simulink model "TRAMI_STEP_AT_vehicle_ver01_R2018b"  (R2018b)
settings: Solver=ode8  StartTime=0  StopTime=end_time  FixedStep=sampling_time  RelTol=1e-3
StartFcn:
  | csvwrite('simstart.csv',1)
StopFcn:
  | csvwrite('simstop.csv',1)
values from neighbouring files (symbols this model uses):
  sampling_time = 0.0025    [METI_TRAMI_Thermal_ver01_Jmaab_PreLoad.m]
undefined symbols (not defined in the file or in its folder): ACC_D_Gain, ACC_I_Gain, ACC_P_Gain, ALT_CNT_ALT_OFF_RPM_HYS_rpm, ALT_CNT_ALT_ON_RPM_HYS_rpm, ALT_CNT_Alter_V_BASE_V, ALT_CNT_Alter_V_Kaisei_V, ALT_CNT_flag_disable_kaisei, ALT_CNT_V_Battely_Kudo_V, ALT_PNT_ALT_GDCurrent_A, ALT_PNT_ALT_GDVolt_V, ALT_PNT_Alter_limit_Current_V_table, ALT_PNT_Alter_limit_Current_V_table_x_rpm, ALT_PNT_Alter_trq_Nm_map, ALT_PNT_Alter_trq_Nm_map_x_rpm, ALT_PNT_Alter_trq_Nm_map_y_Current_A, ALT_PNT_Alter_trq_Nm_map_z_Volt_tgt_V, ALT_PNT_eta_pulley_alt, ALT_PNT_Gain_Alt_v_del, ALT_PNT_ratio_pulley_alt, ALT_PNT_Tau_Alternator_V_tgt_s, ALT_PNT_trq_alter_output_LL_Nm, BK_PNT_Pow_UL, BK_PNT_Tau_brake, Brk_LL, Brk_PGain, Brk_UL, BT_PNT_Lo_Capa_lo_batt_F, BT_PNT_Lo_ocv_SOC_lo_batt_OCV_V_table, BT_PNT_Lo_ocv_SOC_lo_batt_OCV_V_table_x_SOC, BT_PNT_Lo_R_lo_batt_ohm, BT_PNT_Lo_SOC_MAX_lo_batt, BT_PNT_Lo_SOC_MIN_lo_batt, BT_PNT_Lo_SOC_START_lo_batt, BT_PNT_Lo_V_start_ocv, Driver_Brake_Const1, Driver_Brake_Const3, Driver_Brake_Switch_Const2, Driver_Brk_sh, drivmode_ACC, drivmode_CONST, drivmode_GensokuKaisei, drivmode_GensokuRikko, drivmode_STOP, EL_PNT_R_bodyelec_lo_ohm, ENG_CNT_Accel_LL, ENG_CNT_Accel_UL, ENG_CNT_brak_idlestop, ENG_CNT_flag_idle_stop_exe, ENG_CNT_gain_p_per_isc, ENG_CNT_IdleSpeed_Const, ENG_CNT_omg_eng_fuelcut_rpm, ENG_CNT_per_isc_max, ENG_CNT_per_isc_min, ENG_CNT_per_throttle_fuelcut, ENG_CNT_per_throttle_isc_fb, ENG_CNT_Starter_timer_Const_s, ENG_CNT_Throttle_LL, ENG_CNT_Throttle_UL, ENG_CNT_V_car_idlestop_kmph ... (+29)
libraries: METI_Lib_vehicle_model x18, simulink x4, AZAPA_Lib_vehicle_model x1
(part 2 of 2)

== system TRAMI_STEP_AT_vehicle_ver01_R2018b/Vehicle/TR_PNT ==
  note: 転がり抵抗
  note: 並進⇔回転変換
  note: トルク⇔力変換
  note: omg (回転数rad/s) = v (車速m/s) / r (タイヤ半径(m))
  note: M (トルクNm) = F (力(N)） × r (タイヤ半径(m))
  note: 車両を動かす側が正
  note: 車両を動かす側が正
  trq_TR_in_Nm : Inport
  v_VL_PNT_mps : Inport  Port=2
  Constant2 : Constant  Value=1/tire_r
  Product5 : Product  RndMeth=Zero
  Product6 : Product  RndMeth=Zero
  Q_cal1 : METI_Lib_vehicle_model/P_cal  Commented=on  Type_energy=並進運動  Type_output_energy=出力  Power_name=Po_  t_Workspace_Name=TR_PNT_MECK_DN  P_VariableName=Po_TR_PNT_MECK_DN  Across_VariableName=v_TR_PNT_MECK_DN  Throgh_VariableName=F_TR_PNT_MECK_DN
      settings: SourceProductName=The database C:\Users\k-uekata\AppData\Roaming\MathWorks\MATLAB\R2018b\slblocks_master.db is locked, or a table in the database is locked. (database is locked)
  Q_cal2 : METI_Lib_vehicle_model/P_cal  Commented=on  Type_energy=回転運動  Type_output_energy=出力  Power_name=Po_  t_Workspace_Name=TR_PNT_MECK_UP  P_VariableName=Po_TR_PNT_MECK_UP  Across_VariableName=w_TR_PNT_MECK_UP  Throgh_VariableName=tq_TR_PNT_MECK_UP
      settings: SourceProductName=The database C:\Users\k-uekata\AppData\Roaming\MathWorks\MATLAB\R2018b\slblocks_master.db is locked, or a table in the database is locked. (database is locked)
  Sum2 : Sum  Inputs=-+|
  Terminator1 : Terminator  Commented=on
  Terminator2 : Terminator  Commented=on
  cal_roll_resi : METI_Lib_vehicle_model/vehicle_model/cal_roll_resi  Myu_tire=myu  Vehicle_Mass=M  Gravi_acc=g
      settings: SourceProductName=The database C:\Users\k-uekata\AppData\Roaming\MathWorks\MATLAB\R2018b\slblocks_master.db is locked, or a table in the database is locked. (database is locked)
  w_TR_PNT_radps : Outport
  f_TR_PNT_N : Outport  Port=2
  wires:
  Sum2/1 -> f_TR_PNT_N/1  "f_TR_PNT_N"
  cal_roll_resi/1 -> Sum2/1, Q_cal1/2
  Product6/1 -> Sum2/2, Q_cal2/2
  Q_cal1/1 -> Terminator1/1
  Constant2/1 -> Product6/1, Product5/2
  v_VL_PNT_mps/1 -> Product5/1, cal_roll_resi/1, Q_cal1/1, Q_cal2/1
  Q_cal2/1 -> Terminator2/1
  Product5/1 -> w_TR_PNT_radps/1  "w_TR_PNT_radps"
  trq_TR_in_Nm/1 -> Product6/2

== system TRAMI_STEP_AT_vehicle_ver01_R2018b/Vehicle/T_PT_TH_K ==
  From Workspace1 : FromWorkspace  VariableName=T_PT_TH_K  SampleTime=0  OutputAfterFinalValue=Holding final value
  Sum2 : Sum  Inputs=|++
  ℃⇒K : Constant  Value=273.15
  Out1 : Outport
  wires:
  From Workspace1/1 -> Sum2/1
  ℃⇒K/1 -> Sum2/2
  Sum2/1 -> Out1/1

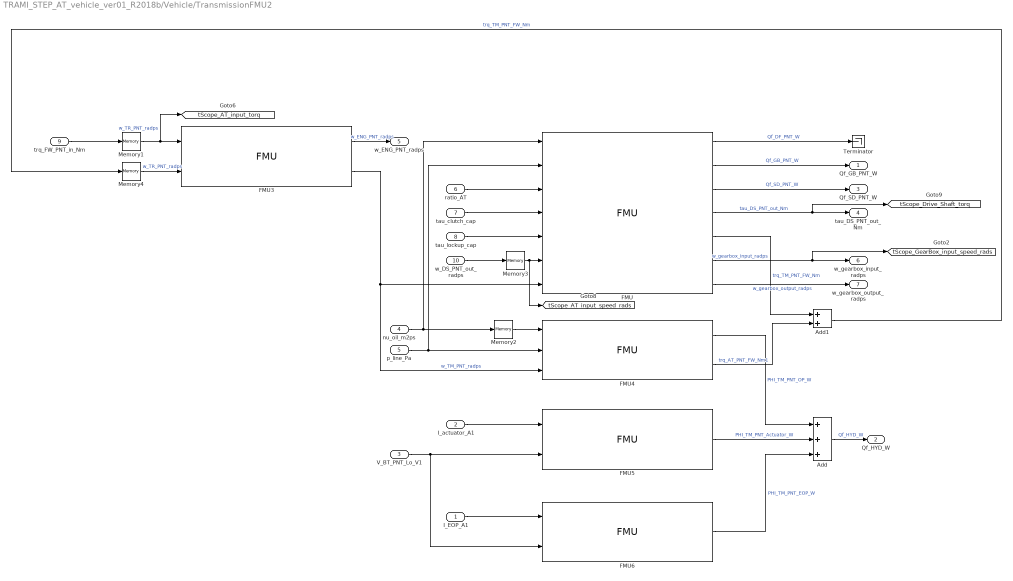
== system TRAMI_STEP_AT_vehicle_ver01_R2018b/Vehicle/TransmissionFMU2 ==
  I_EOP_A1 : Inport
  I_actuator_A1 : Inport  Port=2
  V_BT_PNT_Lo_V1 : Inport  Port=3
  nu_oil_m2ps : Inport  Port=4
  p_line_Pa : Inport  Port=5
  ratio_AT : Inport  Port=6
  tau_clutch_cap : Inport  Port=7
  tau_lockup_cap : Inport  Port=8
  trq_FW_PNT_in_Nm : Inport  Port=9
  w_DS_PNT_out_radps : Inport  Port=10
  Add : Sum  Inputs=+++
  Add1 : Sum
  FMU : FMU  FMUName=AtDsFmu.fmu  FMUMode=CoSimulation  minsamplestep=2.50000000000000000e-02  binfilename=DISABLED  mask(AtDsFmu [Co-Simulation, v2.0]){}
      mask Display: disp('AtDsFmu');
  FMU3 : FMU  FMUName=Flywheel.fmu  FMUMode=CoSimulation  Iwh=4.00000000000000000e-01  minsamplestep=2.50000000000000000e-02  binfilename=DISABLED  mask(Flywheel [Co-Simulation, v2.0]){}
      mask Display: disp('Flywheel');
  FMU4 : FMU  FMUName=OilPump.fmu  FMUMode=CoSimulation  Oil_Viscosity_Breakpoint_2=1.02000000000000000e-05  Oil_Viscosity_Breakpoint_3=1.69000000000000000e-05  Oil_Viscosity_Breakpoint_4=3.12000000000000000e-05  minsamplestep=2.50000000000000000e-02  binfilename=DISABLED  mask(OilPump [Co-Simulation, v2.0]){}
      mask Display: disp('OilPump');
  FMU5 : FMU  FMUName=ActuatorELoss.fmu  FMUMode=CoSimulation  minsamplestep=2.50000000000000000e-02  binfilename=DISABLED  mask(ActuatorELoss [Co-Simulation, v2.0]){}
      mask Display: disp('ActuatorELoss');
  FMU6 : FMU  FMUName=EOPELoss.fmu  FMUMode=CoSimulation  minsamplestep=2.50000000000000000e-02  binfilename=DISABLED  mask(EOPELoss [Co-Simulation, v2.0]){}
      mask Display: disp('EOPELoss');
  Memory{1..4} (4 alike) : Memory
  Terminator : Terminator
  Qf_GB_PNT_W : Outport
  Qf_HYD_W : Outport  Port=2
  Qf_SD_PNT_W : Outport  Port=3
  tau_DS_PNT_out_Nm : Outport  Port=4
  w_ENG_PNT_radps : Outport  Port=5
  w_gearbox_input_radps : Outport  Port=6
  w_gearbox_output_radps : Outport  Port=7
  tag scope: tScope_AT_input_speed_rads=global, tScope_AT_input_torq=global, tScope_Drive_Shaft_torq=global, tScope_GearBox_input_speed_rads=global
  wires:
  FMU3/1 -> w_ENG_PNT_radps/1  "w_ENG_PNT_radps"
  FMU5/1 -> Add/2  "PHI_TM_PNT_Actuator_W"
  FMU6/1 -> Add/3  "PHI_TM_PNT_EOP_W"
  FMU4/1 -> Add/1  "PHI_TM_PNT_OP_W"
  Add/1 -> Qf_HYD_W/1  "Qf_HYD_W"
  FMU4/2 -> Add1/2  "trq_AT_PNT_FW_Nm1"
  I_EOP_A1/1 -> FMU6/1
  I_actuator_A1/1 -> FMU5/1
  V_BT_PNT_Lo_V1/1 -> FMU6/2, FMU5/2
  trq_FW_PNT_in_Nm/1 -> Memory1/1
  p_line_Pa/1 -> FMU/2, FMU4/2
  nu_oil_m2ps/1 -> FMU/1, Memory2/1
  FMU3/2 -> FMU/7, FMU4/3  "w_TM_PNT_radps"
  Add1/1 -> Memory4/1  "trq_TM_PNT_FW_Nm"
  ratio_AT/1 -> FMU/3
  tau_clutch_cap/1 -> FMU/4
  tau_lockup_cap/1 -> FMU/5
  FMU/5 -> Add1/1  "trq_TM_PNT_FW_Nm"
  FMU/1 -> Terminator/1  "Qf_DF_PNT_W"
  FMU/2 -> Qf_GB_PNT_W/1  "Qf_GB_PNT_W"
  FMU/3 -> Qf_SD_PNT_W/1  "Qf_SD_PNT_W"
  FMU/4 -> [tScope_Drive_Shaft_torq], tau_DS_PNT_out_Nm/1  "tau_DS_PNT_out_Nm"
  FMU/6 -> [tScope_GearBox_input_speed_rads], w_gearbox_input_radps/1  "w_gearbox_input_radps"
  FMU/7 -> w_gearbox_output_radps/1  "w_gearbox_output_radps"
  Memory2/1 -> FMU4/1
  Memory1/1 -> [tScope_AT_input_torq], FMU3/1  "w_TR_PNT_radps"
  w_DS_PNT_out_radps/1 -> Memory3/1
  Memory4/1 -> FMU3/2  "w_TR_PNT_radps"
  Memory3/1 -> [tScope_AT_input_speed_rads], FMU/6

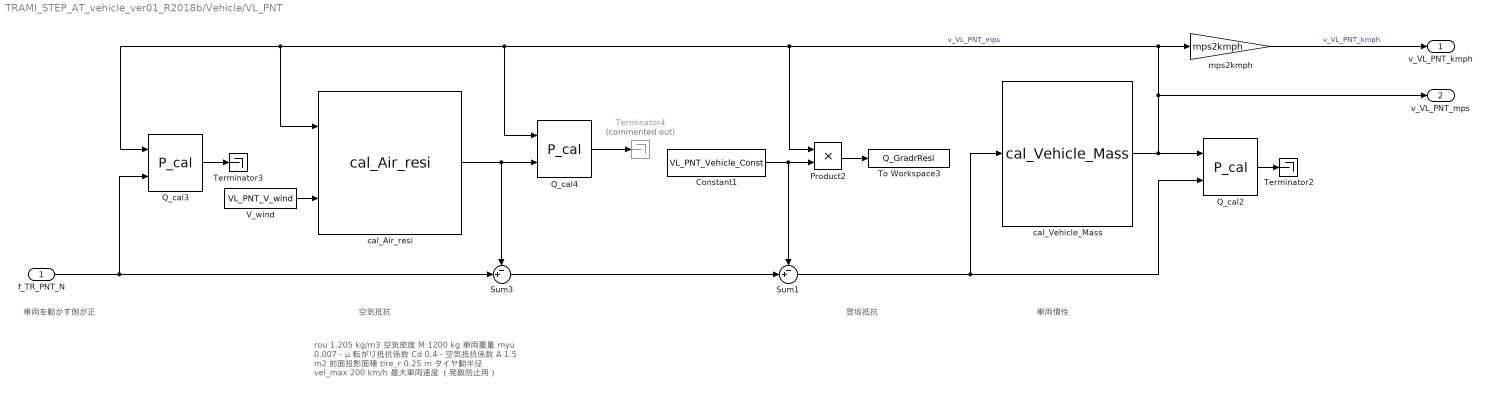
== system TRAMI_STEP_AT_vehicle_ver01_R2018b/Vehicle/VL_PNT ==
  note: rou 1.205 kg/m3 空気密度
      |  M 1200 kg 車両重量
      |  myu 0.007 - μ 転がり抵抗係数
      |  Cd 0.4 - 空気抵抗係数
      |  A 1.5 m2 前面投影面積
      |  tire_r 0.25 m タイヤ動半径
      |  vel_max 200 km/h 最大車両速度 （発散防止用）
  note: 空気抵抗
  note: 車両慣性
  note: 登坂抵抗
  note: 車両を動かす側が正
  f_TR_PNT_N : Inport
  Constant1 : Constant  Value=VL_PNT_Vehicle_Const
  Product2 : Product
  Q_cal2 : METI_Lib_vehicle_model/P_cal  Type_energy=並進運動  Type_output_energy=出力  Power_name=Po_  t_Workspace_Name=VL_PNT_MASS_MECK  P_VariableName=Po_VL_PNT_MASS_MECK  Across_VariableName=v_VL_PNT_MASS_MECK  Throgh_VariableName=F_VL_PNT_MASS_MECK
      settings: SourceProductName=The database C:\Users\k-uekata\AppData\Roaming\MathWorks\MATLAB\R2018b\slblocks_master.db is locked, or a table in the database is locked. (database is locked)
  Q_cal3 : METI_Lib_vehicle_model/P_cal  Type_energy=並進運動  Type_output_energy=出力  Power_name=Po_  t_Workspace_Name=VL_PNT_MECK  P_VariableName=Po_VL_PNT_MECK  Across_VariableName=v_VL_PNT_MECK  Throgh_VariableName=F_VL_PNT_MECK
      settings: SourceProductName=The database C:\Users\k-uekata\AppData\Roaming\MathWorks\MATLAB\R2018b\slblocks_master.db is locked, or a table in the database is locked. (database is locked)
  Q_cal4 : METI_Lib_vehicle_model/P_cal  Type_energy=並進運動  Type_output_energy=損失  Power_name=Pl_  t_Workspace_Name=VL_PNT_Airresi_MECK_LOSS  P_VariableName=Pl_VL_PNT_Airresi_MECK_LOSS  Across_VariableName=v_VL_PNT_Airresi_MECK_LOSS  Throgh_VariableName=F_VL_PNT_Airresi_MECK_LOSS
      settings: SourceProductName=The database C:\Users\k-uekata\AppData\Roaming\MathWorks\MATLAB\R2018b\slblocks_master.db is locked, or a table in the database is locked. (database is locked)
  Sum1 : Sum  Inputs=-+|
  Sum3 : Sum  Inputs=-+|
  Terminator2 : Terminator
  Terminator3 : Terminator
  Terminator4 : Terminator  Commented=on
  To Workspace3 : ToWorkspace  VariableName=Q_GradrResi  SaveFormat=Structure With Time  SampleTime=-1
      settings: Decimation=100
  V_wind : Constant  Value=VL_PNT_V_wind
  cal_Air_resi : METI_Lib_vehicle_model/vehicle_model/cal_Air_resi  Vel_max=vel_max
      settings: SourceProductName=The database C:\Users\k-uekata\AppData\Roaming\MathWorks\MATLAB\R2018b\slblocks_master.db is locked, or a table in the database is locked. (database is locked)
  cal_Vehicle_Mass : METI_Lib_vehicle_model/vehicle_model/cal_Vehicle_Mass  Vehicle_Mass=M
      settings: SourceProductName=The database C:\Users\k-uekata\AppData\Roaming\MathWorks\MATLAB\R2018b\slblocks_master.db is locked, or a table in the database is locked. (database is locked)
  mps2kmph : Gain  Gain=mps2kmph
  v_VL_PNT_kmph : Outport
  v_VL_PNT_mps : Outport  Port=2
  wires:
  Product2/1 -> To Workspace3/1
  Sum3/1 -> Sum1/2
  Sum1/1 -> Q_cal2/2, cal_Vehicle_Mass/1
  cal_Vehicle_Mass/1 -> v_VL_PNT_mps/1, Q_cal3/1, cal_Air_resi/1, Q_cal4/1, Product2/1, mps2kmph/1, Q_cal2/1  "v_VL_PNT_mps"
  cal_Air_resi/1 -> Q_cal4/2, Sum3/1
  V_wind/1 -> cal_Air_resi/2
  Constant1/1 -> Product2/2, Sum1/1
  Q_cal2/1 -> Terminator2/1
  Q_cal3/1 -> Terminator3/1
  Q_cal4/1 -> Terminator4/1
  mps2kmph/1 -> v_VL_PNT_kmph/1  "v_VL_PNT_kmph"
  f_TR_PNT_N/1 -> Sum3/2, Q_cal3/2

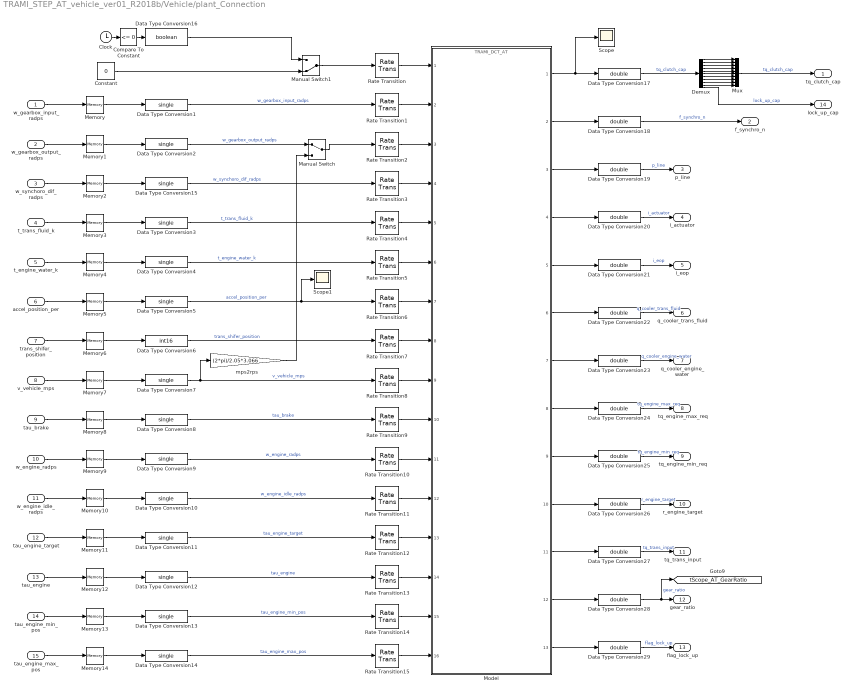
== system TRAMI_STEP_AT_vehicle_ver01_R2018b/Vehicle/plant_Connection ==
  w_gearbox_input_radps : Inport
  w_gearbox_output_radps : Inport  Port=2
  w_synchoro_dif_radps : Inport  Port=3
  t_trans_fluid_k : Inport  Port=4
  t_engine_water_k : Inport  Port=5
  accel_position_per : Inport  Port=6
  trans_shifer_position : Inport  Port=7
  v_vehicle_mps : Inport  Port=8
  tau_brake : Inport  Port=9
  w_engine_radps : Inport  Port=10
  w_engine_idle_radps : Inport  Port=11
  tau_engine_target : Inport  Port=12
  tau_engine : Inport  Port=13
  tau_engine_min_pos : Inport  Port=14
  tau_engine_max_pos : Inport  Port=15
  Clock : Clock
  Compare To Constant : simulink/Logic and Bit Operations/Compare To Constant  relop=<=  const=0  OutDataTypeStr=boolean
  Constant : Constant  Value=0  OutDataTypeStr=boolean
  Data Type Conversion{1..5,7..15} (14 alike) : DataTypeConversion  OutDataTypeStr=single
  Data Type Conversion16 : DataTypeConversion  OutDataTypeStr=boolean
  Data Type Conversion{17..29} (13 alike) : DataTypeConversion  OutDataTypeStr=double
  Data Type Conversion6 : DataTypeConversion  OutDataTypeStr=int16
  Demux : Demux  Outputs=11
  Manual Switch : ManualSwitch
  Manual Switch1 : ManualSwitch  CurrentSetting=0
  Memory{,1..14} (15 alike) : Memory
  Model : ModelReference  ModelNameDialog=TRAMI_DCT_AT.slx  SimulationMode=Normal  ModelReferenceVersion=1.20
  Mux : Mux  Inputs=10
  Rate Transition{,1..15} (16 alike) : RateTransition
  Scope : Scope
  Scope1 : Scope
  mps2rps : Gain  Gain=(2*pi)/2.05*3.066
  tq_clutch_cap : Outport
  f_synchro_n : Outport  Port=2
  p_line : Outport  Port=3
  i_actuator : Outport  Port=4
  i_eop : Outport  Port=5
  q_cooler_trans_fluid : Outport  Port=6
  q_cooler_engine_water : Outport  Port=7
  tq_engine_max_req : Outport  Port=8
  tq_engine_min_req : Outport  Port=9
  r_engine_target : Outport  Port=10
  tq_trans_input : Outport  Port=11
  gear_ratio : Outport  Port=12
  flag_lock_up : Outport  Port=13
  lock_up_cap : Outport  Port=14
  tag scope: tScope_AT_GearRatio=global
  wires:
  Manual Switch1/1 -> Rate Transition/1
  Compare To Constant/1 -> Data Type Conversion16/1
  Clock/1 -> Compare To Constant/1
  Data Type Conversion16/1 -> Manual Switch1/1
  Manual Switch/1 -> Rate Transition2/1
  accel_position_per/1 -> Memory5/1
  Model/10 -> Data Type Conversion26/1
  tau_engine_min_pos/1 -> Memory13/1
  tau_engine/1 -> Memory12/1
  Model/2 -> Data Type Conversion18/1
  w_synchoro_dif_radps/1 -> Memory2/1
  t_trans_fluid_k/1 -> Memory3/1
  Model/4 -> Data Type Conversion20/1
  Model/3 -> Data Type Conversion19/1
  Model/1 -> Scope/1, Data Type Conversion17/1
  Model/11 -> Data Type Conversion27/1
  tau_engine_target/1 -> Memory11/1
  mps2rps/1 -> Manual Switch/2
  v_vehicle_mps/1 -> Memory7/1
  Model/5 -> Data Type Conversion21/1
  Data Type Conversion8/1 -> Rate Transition9/1  "tau_brake"
  trans_shifer_position/1 -> Memory6/1
  Data Type Conversion5/1 -> Rate Transition6/1, Scope1/1  "accel_position_per"
  Model/9 -> Data Type Conversion25/1
  w_gearbox_input_radps/1 -> Memory/1
  Data Type Conversion2/1 -> Manual Switch/1  "w_gearbox_output_radps"
  Data Type Conversion1/1 -> Rate Transition1/1  "w_gearbox_input_radps"
  Data Type Conversion9/1 -> Rate Transition10/1  "w_engine_radps"
  Model/6 -> Data Type Conversion22/1
  w_engine_idle_radps/1 -> Memory10/1
  Data Type Conversion15/1 -> Rate Transition3/1  "w_synchoro_dif_radps"
  Model/13 -> Data Type Conversion29/1
  Data Type Conversion13/1 -> Rate Transition14/1  "tau_engine_min_pos"
  Data Type Conversion14/1 -> Rate Transition15/1  "tau_engine_max_pos"
  Data Type Conversion11/1 -> Rate Transition12/1  "tau_engine_target"
  tau_brake/1 -> Memory8/1
  Data Type Conversion6/1 -> Rate Transition7/1  "trans_shifer_position"
  w_gearbox_output_radps/1 -> Memory1/1
  Constant/1 -> Manual Switch1/2
  t_engine_water_k/1 -> Memory4/1
  Data Type Conversion10/1 -> Rate Transition11/1  "w_engine_idle_radps"
  w_engine_radps/1 -> Memory9/1
  tau_engine_max_pos/1 -> Memory14/1
  Model/12 -> Data Type Conversion28/1
  Model/7 -> Data Type Conversion23/1
  Model/8 -> Data Type Conversion24/1
  Data Type Conversion12/1 -> Rate Transition13/1  "tau_engine"
  Data Type Conversion3/1 -> Rate Transition4/1  "t_trans_fluid_k"
  Data Type Conversion4/1 -> Rate Transition5/1  "t_engine_water_k"
  Data Type Conversion7/1 -> Rate Transition8/1, mps2rps/1  "v_vehicle_mps"
  Mux/1 -> tq_clutch_cap/1  "tq_clutch_cap"
  Data Type Conversion19/1 -> p_line/1  "p_line"
  Data Type Conversion20/1 -> i_actuator/1  "i_actuator"
  Data Type Conversion21/1 -> i_eop/1  "i_eop"
  Data Type Conversion22/1 -> q_cooler_trans_fluid/1  "q_cooler_trans_fluid"
  Data Type Conversion23/1 -> q_cooler_engine_water/1  "q_cooler_engine_water"
  Data Type Conversion24/1 -> tq_engine_max_req/1  "tq_engine_max_req"
  Data Type Conversion25/1 -> tq_engine_min_req/1  "tq_engine_min_req"
  Data Type Conversion26/1 -> r_engine_target/1  "r_engine_target"
  Data Type Conversion27/1 -> tq_trans_input/1  "tq_trans_input"
  Data Type Conversion28/1 -> [tScope_AT_GearRatio], gear_ratio/1  "gear_ratio"
  Memory/1 -> Data Type Conversion1/1
  Memory1/1 -> Data Type Conversion2/1
  Memory2/1 -> Data Type Conversion15/1
  Memory3/1 -> Data Type Conversion3/1
  Memory4/1 -> Data Type Conversion4/1
  Memory5/1 -> Data Type Conversion5/1
  Memory6/1 -> Data Type Conversion6/1
  Memory7/1 -> Data Type Conversion7/1
  Memory8/1 -> Data Type Conversion8/1
  Memory9/1 -> Data Type Conversion9/1
  Memory10/1 -> Data Type Conversion10/1
  Memory11/1 -> Data Type Conversion11/1
  Memory12/1 -> Data Type Conversion12/1
  Memory13/1 -> Data Type Conversion13/1
  Memory14/1 -> Data Type Conversion14/1
  Data Type Conversion18/1 -> f_synchro_n/1  "f_synchro_n"
  Data Type Conversion17/1 -> Demux/1  "tq_clutch_cap"
  Demux/11 -> lock_up_cap/1  "lock_up_cap"
  Demux/1 -> Mux/1
  Demux/2 -> Mux/2
  Demux/3 -> Mux/3
  Demux/4 -> Mux/4
  Demux/5 -> Mux/5
  Demux/6 -> Mux/6
  Demux/7 -> Mux/7
  Demux/8 -> Mux/8
  Demux/9 -> Mux/9
  Demux/10 -> Mux/10
  Rate Transition/1 -> Model/1
  Rate Transition1/1 -> Model/2
  Rate Transition2/1 -> Model/3
  Rate Transition3/1 -> Model/4
  Rate Transition4/1 -> Model/5
  Rate Transition5/1 -> Model/6
  Rate Transition6/1 -> Model/7
  Rate Transition7/1 -> Model/8
  Rate Transition8/1 -> Model/9
  Rate Transition9/1 -> Model/10
  Rate Transition10/1 -> Model/11
  Rate Transition11/1 -> Model/12
  Rate Transition12/1 -> Model/13
  Rate Transition13/1 -> Model/14
  Rate Transition14/1 -> Model/15
  Rate Transition15/1 -> Model/16
  Data Type Conversion29/1 -> flag_lock_up/1  "flag_lock_up"

== system TRAMI_STEP_AT_vehicle_ver01_R2018b/Driver/Caliculate_Opeining_Accel/FB ==
  delta_v_VL_kmph : Inport
  Acc_D_Gain : Gain  Gain=D_Gain
  Acc_I_Gain : Gain  Gain=I_Gain
  Acc_P_Gain : Gain  Gain=P_Gain
  Acc_P_Gain1 : Gain  Gain=P_Gain
  Derivative : Derivative
  Filter : Subsystem  Commented=through
  Integrator : Integrator
  Memory : Memory
  Product1 : Product
  Saturation2 : Saturate  UpperLimit=1  LowerLimit=0
  Sum : Sum  Inputs=+++
  Terminator : Terminator
  FB_open_accel_per : Outport
  wires:
  Filter/1(Out1) -> Product1/2
  Saturation2/1 -> Acc_P_Gain/1
  Acc_P_Gain/1 -> Product1/1
  Sum/1 -> FB_open_accel_per/1
  Derivative/1 -> Acc_D_Gain/1
  Integrator/1 -> Acc_I_Gain/1
  delta_v_VL_kmph/1 -> Memory/1
  Acc_I_Gain/1 -> Sum/3
  Acc_D_Gain/1 -> Sum/2
  Product1/1 -> Sum/1
  Memory/1 -> Saturation2/1, Filter/1(In1), Acc_P_Gain1/1, Integrator/1, Derivative/1
  Acc_P_Gain1/1 -> Terminator/1

== system TRAMI_STEP_AT_vehicle_ver01_R2018b/Driver/Caliculate_Opeining_Accel/FF ==
  note: 速度とパワーでF/B出来るようにモデルを用意しておく
      | 切り替えスイッチを作っておく
  v_VL_PNT_kmph : Inport
  target_v_VL_kmph : Inport  Port=2
  pre_n_eng_rpm : Inport  Port=3
  pre_ratio_DCT : Inport  Port=4
  Air_Resistance : Subsystem
  Cal_M_ENG_jiku2 : Subsystem
  Constant : Constant  Value=0.1
  Constant3 : Constant  Value=tire_r
  Constant4 : Constant  Value=TM_PNT_FD_gear
  Inertial_Resistance : Subsystem
  MinMax : MinMax  Function=max  Inputs=2
  Product8 : Product  Inputs=*/*/  RndMeth=Zero
  Rolling_Resistance : Subsystem
  Sum4 : Sum  Inputs=+++
  Terminator : Terminator
  kmph2mps : Gain  Gain=kmph2mps
  kmph2mps1 : Gain  Gain=kmph2mps
  FF_open_accel_per : Outport
  wires:
  kmph2mps/1 -> Inertial_Resistance/1(V_tgt), Rolling_Resistance/1(V_tgt), Air_Resistance/1(V_tgt)
  target_v_VL_kmph/1 -> kmph2mps/1
  Sum4/1 -> Product8/1
  Constant4/1 -> Product8/2
  Constant3/1 -> Product8/3
  Air_Resistance/1(F_air_resi) -> Sum4/2
  Rolling_Resistance/1(F_rollresi) -> Sum4/3
  Inertial_Resistance/1(F_Inertia) -> Sum4/1
  pre_ratio_DCT/1 -> MinMax/2
  v_VL_PNT_kmph/1 -> kmph2mps1/1
  kmph2mps1/1 -> Terminator/1
  Cal_M_ENG_jiku2/1(FF_open_accel_per) -> FF_open_accel_per/1
  Product8/1 -> Cal_M_ENG_jiku2/1(FF_trq_accel_Nm)  "FF_trq_accel_Nm"
  pre_n_eng_rpm/1 -> Cal_M_ENG_jiku2/2(pre_n_eng_rpm)
  Constant/1 -> MinMax/1
  MinMax/1 -> Product8/4

== system TRAMI_STEP_AT_vehicle_ver01_R2018b/Vehicle/ALT_PNT/Subsystem ==
  note: V_ALT_PNT
  note: オルタ要求トルク上限/下限ガード処理追加
      | (低回転数、低電流時に要求トルクが過大となるのを防止するため
      |  :マップの外挿方法が線形となっていることが原因)
  target_volt_ALT_V : Inport
  w_ROT_slavepulley12 : Inport  Port=2
  volt_BT_PNT_Lo_V : Inport  Port=3
  Constant1 : Constant  Value=ALT_PNT_ALT_GDCurrent_A
  Constant2 : Constant  Value=ALT_PNT_ALT_GDVolt_V
  I_alt_cal : Subsystem
  Torque_Guard : Subsystem
  Transfer Fcn1 : TransferFcn  Denominator=|
      | [ALT_PNT_Tau_Alternator_trq_Nm
      |  1]
  omg2rpm : Gain  Gain=radpsec2rpm
  current_ALT_PNT_A : Outport
  trq_trqsource : Outport  Port=2
  wires:
  I_alt_cal/1(I_alt) -> Torque_Guard/1(current_ALT_PNT_A), current_ALT_PNT_A/1  "current_ALT_PNT_A"
  target_volt_ALT_V/1 -> I_alt_cal/1(target_volt_ALT_V)
  volt_BT_PNT_Lo_V/1 -> Torque_Guard/2(V_ALT_PNT), I_alt_cal/2(volt_BT_PNT_Lo_V)
  Transfer Fcn1/1 -> trq_trqsource/1
  omg2rpm/1 -> Torque_Guard/3(n_ROT_slavepulley12_rpm), I_alt_cal/3(rpm_alt)  "n_ROT_slavepulley12_rpm"
  w_ROT_slavepulley12/1 -> omg2rpm/1
  Constant1/1 -> Torque_Guard/4(ALT_GDCurrent)
  Constant2/1 -> Torque_Guard/5(ALT_GDVolt)
  Torque_Guard/1(trq_trqsource) -> Transfer Fcn1/1

== system TRAMI_STEP_AT_vehicle_ver01_R2018b/Vehicle/ALT_PNT/pulley_slave ==
  note: プーリー比
  note: プーリー効率
  w_ENG_PNT_radps : Inport
  trq_slavepulley12 : Inport  Port=2
  Goto3 : Goto  Commented=on  GotoTag=tScope_pulley1Loss  TagVisibility=global
  P_cal : AZAPA_Lib_vehicle_model/P_cal  Commented=on  Type_energy=並進運動  Type_output_energy=出力  Power_name=Po_  t_Workspace_Name=MOTOR_MECK  P_VariableName=Po_MOTOR_MECK  Across_VariableName=v_MOTOR_MECK  Throgh_VariableName=F_MOTOR_MECK
  Product : Product  RndMeth=Zero
  Product1 : Product  RndMeth=Zero
  eta_cal2 : METI_Lib_vehicle_model/eta_cal2  SystemSampleTime=-1
      settings: SourceProductName=The database C:\Users\k-uekata\AppData\Roaming\MathWorks\MATLAB\R2018b\slblocks_master.db is locked, or a table in the database is locked. (database is locked)
  eta_pulley : Constant  Value=ALT_PNT_eta_pulley_alt
  ratio_pulley : Constant  Value=ALT_PNT_ratio_pulley_alt
  trq_slavepulley11 : Outport
  w_slavepulley12 : Outport  Port=2
  wires:
  eta_cal2/1 -> P_cal/2
  P_cal/1 -> Goto3/1
  w_ENG_PNT_radps/1 -> P_cal/1, Product1/1
  eta_cal2/2 -> trq_slavepulley11/1
  trq_slavepulley12/1 -> Product/2
  eta_pulley/1 -> eta_cal2/1
  Product1/1 -> w_slavepulley12/1
  ratio_pulley/1 -> Product/1, Product1/2
  Product/1 -> eta_cal2/2

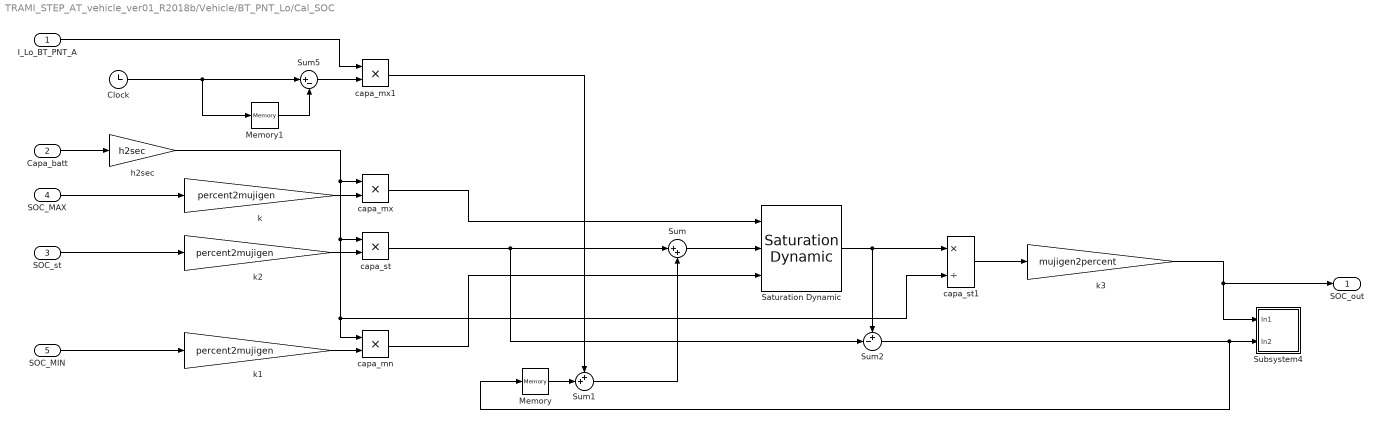
== system TRAMI_STEP_AT_vehicle_ver01_R2018b/Vehicle/BT_PNT_Lo/Cal_SOC ==
  I_Lo_BT_PNT_A : Inport
  Capa_batt : Inport  Port=2
  SOC_st : Inport  Port=3
  SOC_MAX : Inport  Port=4
  SOC_MIN : Inport  Port=5
  Clock : Clock
  Memory : Memory
  Memory1 : Memory
  Saturation Dynamic : simulink/Discontinuities/Saturation Dynamic  OutMin=[]  OutMax=[]  OutDataTypeStr=Inherit: Same as second input  OutDataType=fixdt(1, 16)  OutScaling=2^-10  DoSatur=off
  Subsystem4 : Subsystem  mask{SOC=SOC_LoBat, VariableName=Asec_LoBat}
      mask prompts: SOC "バッテリSOC"; VariableName "バッテリ容量変化量(Asec)"
  Sum : Sum  Inputs=|++
  Sum1 : Sum  Inputs=++|
  Sum2 : Sum  Inputs=+-|
  Sum5 : Sum  Inputs=|+-
  capa_mn : Product  RndMeth=Zero
  capa_mx : Product  RndMeth=Zero
  capa_mx1 : Product  RndMeth=Zero
  capa_st : Product  RndMeth=Zero
  capa_st1 : Product  Inputs=*/  RndMeth=Zero
  h2sec : Gain  Gain=h2sec
  k : Gain  Gain=percent2mujigen
  k1 : Gain  Gain=percent2mujigen
  k2 : Gain  Gain=percent2mujigen
  k3 : Gain  Gain=mujigen2percent
  SOC_out : Outport
  wires:
  Sum5/1 -> capa_mx1/2
  Memory1/1 -> Sum5/2
  Sum/1 -> Saturation Dynamic/2
  Clock/1 -> Sum5/1, Memory1/1
  capa_mx1/1 -> Sum1/1
  k3/1 -> Subsystem4/1(In1), SOC_out/1
  Sum1/1 -> Sum/2
  Memory/1 -> Sum1/2
  k2/1 -> capa_st/2
  k1/1 -> capa_mn/2
  k/1 -> capa_mx/2
  capa_st/1 -> Sum2/2, Sum/1
  Saturation Dynamic/1 -> Sum2/1, capa_st1/1
  capa_mx/1 -> Saturation Dynamic/1
  capa_mn/1 -> Saturation Dynamic/3
  capa_st1/1 -> k3/1
  h2sec/1 -> capa_mn/1, capa_st1/2, capa_st/1, capa_mx/1
  SOC_MIN/1 -> k1/1
  SOC_MAX/1 -> k/1
  SOC_st/1 -> k2/1
  Capa_batt/1 -> h2sec/1
  I_Lo_BT_PNT_A/1 -> capa_mx1/1
  Sum2/1 -> Memory/1, Subsystem4/2(In2)

== system TRAMI_STEP_AT_vehicle_ver01_R2018b/Vehicle/BT_PNT_Lo/Subsystem ==
  I_BT_PNT_Lo_A : Inport
  Divide : Product
  Resistivity : Constant  Value=BT_PNT_Lo_R_lo_batt_ohm
  Sum : Sum  Inputs=|++
  Transfer Fcn : TransferFcn  Numerator=[0.01]  Denominator=[0.1 1]
  V_BT_PNT_Lo_V : Outport
  wires:
  Resistivity/1 -> Divide/2
  Divide/1 -> Sum/1
  I_BT_PNT_Lo_A/1 -> Divide/1, Transfer Fcn/1
  Sum/1 -> V_BT_PNT_Lo_V/1
  Transfer Fcn/1 -> Sum/2

== system TRAMI_STEP_AT_vehicle_ver01_R2018b/Vehicle/ENG_CNT/Caliculate_Idle_Speed ==
  note: 目標アイドル回転数
  note: ○目標回転数に対するP制御
  note: 補機負荷やNDの時の負荷によるアイドル安定化処理を入れる
      | パワーデマンドで締結
  per_throttle_base : Inport
  n_eng_rpm : Inport  Port=2
  flag_cutch_open : Inport  Port=3
  flag_IdleStop : Inport  Port=4
  IdleSpeed : Constant  Value=ENG_CNT_IdleSpeed_Const
  Subsystem : Subsystem
  Subsystem1 : Subsystem
  Subtract : Sum  Inputs=+-
  per_isc_[%] : Outport
  tag scope: ENG_CNT_IdleSpeed_Const=global
  wires:
  IdleSpeed/1 -> Subsystem1/1(omg_tgt_idle), Subtract/1, [ENG_CNT_IdleSpeed_Const]
  n_eng_rpm/1 -> Subsystem1/2(n_eng_rpm), Subtract/2
  Subtract/1 -> Subsystem/1(del_omg_engine)
  per_throttle_base/1 -> Subsystem1/3(per_throttle_base)
  flag_cutch_open/1 -> Subsystem1/4(flag_cutch_open)
  Subsystem1/1(flag_idle_fb) -> Subsystem/2(flag_idle_fb)
  flag_IdleStop/1 -> Subsystem1/5(flag_IdleStop)
  Subsystem/1(per_isc_[%]) -> per_isc_[%]/1

== system TRAMI_STEP_AT_vehicle_ver01_R2018b/Vehicle/ENG_CNT/Set_Fuel_Cut ==
  note: ○減速時のフューエルカット条件
      | 　・停車中でない
      | 　・回転数がある回転数以上
      | 　・アクセル開度がOFF
  v_vehicle : Inport
  n_eng_rpm : Inport  Port=2
  per_throttle_base : Inport  Port=3
  Constant1 : Constant  Value=ENG_CNT_V_vhicle_fuelcut_kmph
  Constant4 : Constant  Value=ENG_CNT_omg_eng_fuelcut_rpm
  Constant6 : Constant  Value=ENG_CNT_per_throttle_fuelcut
  Logical Operator : Logic  Inputs=3  AllPortsSameDT=off  OutDataTypeStr=boolean
  Relational Operator1 : RelationalOperator  Operator=<=  OutDataTypeStr=boolean  RndMeth=Nearest
  Relational Operator2 : RelationalOperator  OutDataTypeStr=boolean  RndMeth=Nearest
  Relational Operator3 : RelationalOperator  OutDataTypeStr=boolean  RndMeth=Nearest
  flag_fuelcut : Outport
  wires:
  n_eng_rpm/1 -> Relational Operator2/1
  per_throttle_base/1 -> Relational Operator1/1
  Constant6/1 -> Relational Operator1/2
  Relational Operator1/1 -> Logical Operator/3
  Relational Operator2/1 -> Logical Operator/2
  Logical Operator/1 -> flag_fuelcut/1
  Constant1/1 -> Relational Operator3/2
  v_vehicle/1 -> Relational Operator3/1
  Relational Operator3/1 -> Logical Operator/1
  Constant4/1 -> Relational Operator2/2

== system TRAMI_STEP_AT_vehicle_ver01_R2018b/Vehicle/ENG_CNT/Set_Idle_Stop ==
  note: ○アイドリングストップ制御
      | 　停車時＋ブレーキを踏んでいるとき、アイドリングストップ
  v_vehicle : Inport
  per_brake : Inport  Port=2
  Constant : Constant  Value=ENG_CNT_V_car_idlestop_kmph
  Constant1 : Constant  Value=ENG_CNT_brak_idlestop
  Constant2 : Constant  Value=ENG_CNT_flag_idle_stop_exe
  Logical Operator : Logic  Inputs=3  AllPortsSameDT=off  OutDataTypeStr=boolean
  Relational Operator : RelationalOperator  Operator=<  OutDataTypeStr=boolean  RndMeth=Nearest
  Relational Operator1 : RelationalOperator  OutDataTypeStr=boolean  RndMeth=Nearest
  flag_IdleStop : Outport
  wires:
  Relational Operator/1 -> Logical Operator/2
  Logical Operator/1 -> flag_IdleStop/1
  v_vehicle/1 -> Relational Operator/1
  per_brake/1 -> Relational Operator1/1
  Constant/1 -> Relational Operator/2
  Constant1/1 -> Relational Operator1/2
  Relational Operator1/1 -> Logical Operator/3
  Constant2/1 -> Logical Operator/1

== system TRAMI_STEP_AT_vehicle_ver01_R2018b/Vehicle/ENG_CNT/Starter ==
  note: サンプリング時間
  note: 時間リセット
  note: アイドリングフラグがON→OFFに
      | 切り替わり時スターターON開始
  note: スタータ開始時間
  note: スタータ開始時間から
      | ある時間超えたらOFF
  note: アイドリングフラグがON→OFFに切り替わり時スターターON開始.ある時間を超えたらOFF
  flag_idlestop : Inport
  n_eng_rpm : Inport  Port=2
  Constant2 : Constant  Value=ENG_CNT_Starter_timer_Const_s
  Constant4 : Constant  Value=sampling_time
  Constant5 : Constant  Value=0
  Constant6 : Constant  Value=OFF
  Constant7 : Constant  Value=ON
  IdleSpeed : Constant  Value=ENG_CNT_IdleSpeed_Const/2
  Logical Operator : Logic  Inputs=3  AllPortsSameDT=off  OutDataTypeStr=boolean
  Logical Operator1 : Logic  Operator=NOT  AllPortsSameDT=off  OutDataTypeStr=boolean
  Memory : Memory  InitialCondition=1000
  Memory1 : Memory  InheritSampleTime=on
  Relational Operator1 : RelationalOperator  Operator=<=  OutDataTypeStr=boolean  RndMeth=Nearest
  Relational Operator2 : RelationalOperator  Operator=<  OutDataTypeStr=boolean  RndMeth=Nearest
  Sum5 : Sum  Inputs=|++
  Switch3 : Switch  Criteria=u2 > Threshold  Threshold=0.5
  Switch4 : Switch  Criteria=u2 > Threshold  Threshold=0.5
  flag_ON_Starter : Outport
  wires:
  Switch4/1 -> flag_ON_Starter/1
  Memory/1 -> Sum5/2
  Constant4/1 -> Sum5/1
  Constant5/1 -> Switch3/1
  Sum5/1 -> Switch3/3
  Switch3/1 -> Relational Operator1/1, Memory/1
  Memory1/1 -> Logical Operator/2
  Logical Operator1/1 -> Logical Operator/1
  flag_idlestop/1 -> Memory1/1, Logical Operator1/1
  Logical Operator/1 -> Switch3/2
  Constant2/1 -> Relational Operator1/2
  Relational Operator1/1 -> Switch4/2
  Constant7/1 -> Switch4/1
  Constant6/1 -> Switch4/3
  n_eng_rpm/1 -> Relational Operator2/1
  IdleSpeed/1 -> Relational Operator2/2
  Relational Operator2/1 -> Logical Operator/3

== system TRAMI_STEP_AT_vehicle_ver01_R2018b/Vehicle/ENG_PNT/Cal_FuelComsunption ==
  w_ENG_PNT_radps : Inport
  trq_ENG : Inport  Port=2
  flag_fuelcut : Inport  Port=3
  flag_IdleStop : Inport  Port=4
  timing_ignition : Inport  Port=5
  1-D Lookup Table1 : Lookup_n-D  NumberOfTableDimensions=1  BreakpointsForDimension1=ENG_PNT_trq_fluc_Nm_table_x_spk_tim  Table=ENG_PNT_trq_fluc_Nm_table  RndMeth=Simplest  InputSameDT=on
  Map_FuelRate : Lookup_n-D  BreakpointsForDimension1=ENG_PNT_FuelCon_gps_map_y_trq_Nm  BreakpointsForDimension2=ENG_PNT_FuelCon_gps_map_x_pri_rpm  Table=ENG_PNT_FuelCon_gps_map  RndMeth=Simplest  InputSameDT=on
  Not_cal1 : Subsystem
  Not_cal2 : Subsystem
  Product : Product  Inputs=3  RndMeth=Zero
  Product1 : Product  Inputs=*/  RndMeth=Zero
  radpsec2rpm : Gain  Gain=radpsec2rpm
  FuelComsunption : Outport
  wires:
  trq_ENG/1 -> Product1/1
  radpsec2rpm/1 -> Map_FuelRate/2
  w_ENG_PNT_radps/1 -> radpsec2rpm/1
  Product/1 -> FuelComsunption/1
  Not_cal2/1(Out1) -> Product/3
  Not_cal1/1(Out1) -> Product/2
  flag_fuelcut/1 -> Not_cal1/1(In1)
  flag_IdleStop/1 -> Not_cal2/1(In1)
  timing_ignition/1 -> 1-D Lookup Table1/1
  1-D Lookup Table1/1 -> Product1/2
  Product1/1 -> Map_FuelRate/1
  Map_FuelRate/1 -> Product/1

== system TRAMI_STEP_AT_vehicle_ver01_R2018b/Vehicle/ENG_PNT/Cal_trq_ENG_jiku ==
  note: エンジン軸トルクマップ
  open_throttle_per : Inport
  flag_fuelcut : Inport  Port=2
  flag_IdleStop : Inport  Port=3
  timing_ignition : Inport  Port=4
  w_ENG_PNT_radps : Inport  Port=5
  1-D Lookup Table : Lookup_n-D  NumberOfTableDimensions=1  BreakpointsForDimension1=ENG_PNT_trq_fluc_Nm_table_x_spk_tim  Table=ENG_PNT_trq_fluc_Nm_table  RndMeth=Simplest  InputSameDT=on
  2-D Lookup Table : Lookup_n-D  BreakpointsForDimension1=ENG_PNT_trq_Nm_map_y_throttle  BreakpointsForDimension2=ENG_PNT_trq_Nm_map_x_rpm  Table=ENG_PNT_trq_Nm_map  ExtrapMethod=Clip  UseLastTableValue=on  RndMeth=Simplest  InputSameDT=on
  Model Info : simulink/Model-Wide Utilities/Model Info  Frame=on  DisplayStringWithTags=|  HorizontalTextAlignment=Left  LeftAlignmentValue=0.02
      | 【注記】
      | ・燃料カット時はスロットル開度を0としてエンジンフリクションを付加
      | ・点火タイミングによるトルク変動を想定
      | ・エンジン軸トルクマップの使用
  Not_cal : Subsystem
  Not_cal1 : Subsystem
  Product : Product  RndMeth=Zero
  Product1 : Product  RndMeth=Zero
  Product2 : Product  RndMeth=Zero
  Saturation : Saturate  UpperLimit=ENG_CNT_Throttle_UL  LowerLimit=ENG_CNT_Throttle_LL
  radpsec2rpm : Gain  Gain=radpsec2rpm
  trq_ENG_PNT_Nm : Outport
  wires:
  w_ENG_PNT_radps/1 -> radpsec2rpm/1
  open_throttle_per/1 -> Product/1
  Saturation/1 -> 2-D Lookup Table/1
  radpsec2rpm/1 -> 2-D Lookup Table/2
  timing_ignition/1 -> 1-D Lookup Table/1
  1-D Lookup Table/1 -> Product1/2
  Product/1 -> Saturation/1
  Product2/1 -> Product/2
  flag_fuelcut/1 -> Not_cal/1(In1)
  Not_cal/1(Out1) -> Product2/1
  flag_IdleStop/1 -> Not_cal1/1(In1)
  Not_cal1/1(Out1) -> Product2/2
  Product1/1 -> trq_ENG_PNT_Nm/1  "trq_ENG_PNT_Nm"
  2-D Lookup Table/1 -> Product1/1

== system TRAMI_STEP_AT_vehicle_ver01_R2018b/Vehicle/TM Thermal/ENG ==
  Qf_case_ENG_W : Inport
      settings: AttributesFormatString=|
      | %<Tag>
      | Priority=<%<Priority>>
  Qf_SD_ENG_W : Inport  Port=2
      settings: AttributesFormatString=|
      | %<Tag>
      | Priority=<%<Priority>>
  From Workspace1 : FromWorkspace  VariableName=T_ENG_K  SampleTime=0  OutputAfterFinalValue=Holding final value
  Sum : Sum  Inputs=|++
  Terminator : Terminator
  Terminator1 : Terminator
  ℃⇒K : Constant  Value=273.15
  T_ENG_K : Outport
      settings: AttributesFormatString=|
      | %<Tag>
      | Priority=<%<Priority>>
  wires:
  Qf_SD_ENG_W/1 -> Terminator/1
  Qf_case_ENG_W/1 -> Terminator1/1
  From Workspace1/1 -> Sum/1
  ℃⇒K/1 -> Sum/2
  Sum/1 -> T_ENG_K/1

== system TRAMI_STEP_AT_vehicle_ver01_R2018b/Vehicle/TM Thermal/PT_TH ==
  Qf_cooler_PT_TH_W : Inport
      settings: AttributesFormatString=|
      | %<Tag>
      | Priority=<%<Priority>>
  From Workspace1 : FromWorkspace  VariableName=T_PT_TH_K  SampleTime=0  OutputAfterFinalValue=Holding final value
  Sum : Sum  Inputs=|++
  Terminator : Terminator
  ℃⇒K : Constant  Value=273.15
  T_PT_TH_K : Outport
      settings: AttributesFormatString=|
      | %<Tag>
      | Priority=<%<Priority>>
  wires:
  Qf_cooler_PT_TH_W/1 -> Terminator/1
  ℃⇒K/1 -> Sum/2
  From Workspace1/1 -> Sum/1
  Sum/1 -> T_PT_TH_K/1

== system TRAMI_STEP_AT_vehicle_ver01_R2018b/Vehicle/TM Thermal/air ==
  Qf_case_air_W : Inport
      settings: AttributesFormatString=|
      | %<Tag>
      | Priority=<%<Priority>>
  From Workspace1 : FromWorkspace  VariableName=T_air_K  SampleTime=0  OutputAfterFinalValue=Holding final value
  Sum : Sum  Inputs=|++
  Terminator : Terminator
  ℃⇒K : Constant  Value=273.15
  T_air_K : Outport
      settings: AttributesFormatString=|
      | %<Tag>
      | Priority=<%<Priority>>
  wires:
  Qf_case_air_W/1 -> Terminator/1
  From Workspace1/1 -> Sum/1
  ℃⇒K/1 -> Sum/2
  Sum/1 -> T_air_K/1

== system TRAMI_STEP_AT_vehicle_ver01_R2018b/Driver/Caliculate_Opeining_Accel/FB/Filter ==
  In1 : Inport
  Gain3 : Gain  Gain=10
  Gain4 : Gain  Gain=0.1
  Rounding Function : Rounding  Operator=round
  Out1 : Outport
  wires:
  Rounding Function/1 -> Gain4/1
  In1/1 -> Gain3/1
  Gain3/1 -> Rounding Function/1
  Gain4/1 -> Out1/1

== system TRAMI_STEP_AT_vehicle_ver01_R2018b/Driver/Caliculate_Opeining_Accel/FF/Air_Resistance ==
  V_tgt : Inport
  V_wind : Constant  Value=VL_PNT_V_wind
  cal_Air_resi1 : METI_Lib_vehicle_model/vehicle_model/cal_Air_resi  Vel_max=200
      settings: SourceProductName=The database C:\Users\k-uekata\AppData\Roaming\MathWorks\MATLAB\R2018b\slblocks_master.db is locked, or a table in the database is locked. (database is locked)
  F_air_resi : Outport
  wires:
  V_tgt/1 -> cal_Air_resi1/1
  V_wind/1 -> cal_Air_resi1/2
  cal_Air_resi1/1 -> F_air_resi/1

== system TRAMI_STEP_AT_vehicle_ver01_R2018b/Driver/Caliculate_Opeining_Accel/FF/Cal_M_ENG_jiku2 ==
  note: 軸トルクマップ
  FF_trq_accel_Nm : Inport
  pre_n_eng_rpm : Inport  Port=2
  2-D Lookup Table : Lookup_n-D  BreakpointsForDimension1=ENG_trq_rev  BreakpointsForDimension2=ENG_rpm  Table=ENG_throttle_rev  ExtrapMethod=Clip  UseLastTableValue=on  RndMeth=Simplest  InputSameDT=on
  2-D Lookup Table1 : Lookup_n-D  BreakpointsForDimension1=ENG_PNT_trq_Nm_map_y_throttle  BreakpointsForDimension2=ENG_PNT_trq_Nm_map_x_rpm  Table=ENG_PNT_trq_Nm_map  ExtrapMethod=Clip  UseLastTableValue=on  RndMeth=Simplest  InputSameDT=on
  Constant : Constant  Value=0
  Subsystem : Subsystem
  Sum : Sum  Inputs=|++
  FF_open_accel_per : Outport
  wires:
  FF_trq_accel_Nm/1 -> Sum/1
  2-D Lookup Table/1 -> Subsystem/1(In1)
  pre_n_eng_rpm/1 -> 2-D Lookup Table/2, 2-D Lookup Table1/2
  Constant/1 -> 2-D Lookup Table1/1
  Sum/1 -> 2-D Lookup Table/1
  2-D Lookup Table1/1 -> Sum/2
  Subsystem/1(Out1) -> FF_open_accel_per/1

== system TRAMI_STEP_AT_vehicle_ver01_R2018b/Driver/Caliculate_Opeining_Accel/FF/Inertial_Resistance ==
  V_tgt : Inport
  Constant : Constant  Value=M
  Derivative : Derivative
  Divide : Product  OutDataTypeStr=Inherit: Same as first input
  F_Inertia : Outport
  wires:
  Constant/1 -> Divide/2
  Derivative/1 -> Divide/1
  Divide/1 -> F_Inertia/1
  V_tgt/1 -> Derivative/1

== system TRAMI_STEP_AT_vehicle_ver01_R2018b/Driver/Caliculate_Opeining_Accel/FF/Rolling_Resistance ==
  note: 20151211修正
      |
      | 空気抵抗と表現を統一する、ため
      | -1のGainを削除
  V_tgt : Inport
  cal_roll_resi1 : METI_Lib_vehicle_model/vehicle_model/cal_roll_resi  Myu_tire=myu  Vehicle_Mass=M  Gravi_acc=g
      settings: SourceProductName=The database C:\Users\k-uekata\AppData\Roaming\MathWorks\MATLAB\R2018b\slblocks_master.db is locked, or a table in the database is locked. (database is locked)
  F_rollresi : Outport
  wires:
  V_tgt/1 -> cal_roll_resi1/1
  cal_roll_resi1/1 -> F_rollresi/1

== system TRAMI_STEP_AT_vehicle_ver01_R2018b/Vehicle/ALT_PNT/Subsystem/I_alt_cal ==
  target_volt_ALT_V : Inport
  volt_BT_PNT_Lo_V : Inport  Port=2
  rpm_alt : Inport  Port=3
  Add : Sum
  Cal_I_alt_P_control : Subsystem
  Cal_I_alt_base : Subsystem
  Constant : Constant  Value=12
  Constant4 : Constant  Value=0
  Limit_Current_Max : Lookup_n-D  NumberOfTableDimensions=1  BreakpointsForDimension1=ALT_PNT_Alter_limit_Current_V_table_x_rpm  Table=ALT_PNT_Alter_limit_Current_V_table  ExtrapMethod=Clip  UseLastTableValue=on  RndMeth=Simplest  InputSameDT=on
  MinMax2 : MinMax  Function=max  Inputs=2
  Sum1 : Sum  Inputs=|+-
  Sum2 : Sum  Inputs=-+|
  電圧比較 : MinMax  Inputs=2
  I_alt : Outport
  wires:
  target_volt_ALT_V/1 -> Sum1/1, Sum2/2
  volt_BT_PNT_Lo_V/1 -> Sum2/1
  rpm_alt/1 -> Limit_Current_Max/1
  Constant4/1 -> MinMax2/2
  Limit_Current_Max/1 -> MinMax2/1  "I_limit_ALT"
  電圧比較/1 -> I_alt/1
  Add/1 -> 電圧比較/2
  Sum2/1 -> Cal_I_alt_P_control/1(V_delt_tgt)
  MinMax2/1 -> 電圧比較/1
  Constant/1 -> Sum1/2
  Sum1/1 -> Cal_I_alt_base/1(V_delt_tgt)
  Cal_I_alt_P_control/1(I_alt_base) -> Add/1
  Cal_I_alt_base/1(I_alt_base) -> Add/2

== system TRAMI_STEP_AT_vehicle_ver01_R2018b/Vehicle/ALT_PNT/Subsystem/Torque_Guard ==
  current_ALT_PNT_A : Inport
  V_ALT_PNT : Inport  Port=2
  n_ROT_slavepulley12_rpm : Inport  Port=3
  ALT_GDCurrent : Inport  Port=4
  ALT_GDVolt : Inport  Port=5
  Caliculate_Axes_Torque1 : Lookup_n-D  NumberOfTableDimensions=3  BreakpointsForDimension1=ALT_PNT_Alter_trq_Nm_map_x_rpm  BreakpointsForDimension2=ALT_PNT_Alter_trq_Nm_map_y_Current_A  BreakpointsForDimension3=ALT_PNT_Alter_trq_Nm_map_z_Volt_tgt_V  Table=ALT_PNT_Alter_trq_Nm_map  RndMeth=Simplest  InputSameDT=on
  Caliculate_Axes_Torque2 : Lookup_n-D  NumberOfTableDimensions=3  BreakpointsForDimension1=ALT_PNT_Alter_trq_Nm_map_x_rpm  BreakpointsForDimension2=ALT_PNT_Alter_trq_Nm_map_y_Current_A  BreakpointsForDimension3=ALT_PNT_Alter_trq_Nm_map_z_Volt_tgt_V  Table=ALT_PNT_Alter_trq_Nm_map  RndMeth=Simplest  InputSameDT=on
  Constant3 : Constant  Value=ALT_PNT_trq_alter_output_LL_Nm
  MinMax : MinMax  Inputs=2
  MinMax1 : MinMax  Function=max  Inputs=2
  trq_trqsource : Outport
  wires:
  ALT_GDCurrent/1 -> Caliculate_Axes_Torque2/2
  Caliculate_Axes_Torque2/1 -> MinMax/2
  MinMax/1 -> MinMax1/1
  Caliculate_Axes_Torque1/1 -> MinMax/1
  Constant3/1 -> MinMax1/2
  ALT_GDVolt/1 -> Caliculate_Axes_Torque2/3
  MinMax1/1 -> trq_trqsource/1
  V_ALT_PNT/1 -> Caliculate_Axes_Torque1/3
  current_ALT_PNT_A/1 -> Caliculate_Axes_Torque1/2
  n_ROT_slavepulley12_rpm/1 -> Caliculate_Axes_Torque2/1, Caliculate_Axes_Torque1/1

== system TRAMI_STEP_AT_vehicle_ver01_R2018b/Vehicle/BT_PNT_Lo/Cal_SOC/Subsystem4 ==
  In1 : Inport
  In2 : Inport  Port=2
  To Workspace : ToWorkspace  VariableName=SOC_LoBat  SampleTime=-1
      settings: Decimation=num_tws_mabiki
  To Workspace1 : ToWorkspace  VariableName=Asec_LoBat  SampleTime=-1
      settings: Decimation=num_tws_mabiki
  wires:
  In1/1 -> To Workspace/1
  In2/1 -> To Workspace1/1

== system TRAMI_STEP_AT_vehicle_ver01_R2018b/Vehicle/ENG_CNT/Caliculate_Idle_Speed/Subsystem ==
  del_omg_engine : Inport
  flag_idle_fb : Inport  Port=2
  Gain : Gain  Gain=ENG_CNT_gain_p_per_isc
  Logical Operator1 : Logic  Operator=NOT  AllPortsSameDT=off  OutDataTypeStr=boolean
  Memory : Memory  InitialCondition=4
  Saturation : Saturate  UpperLimit=ENG_CNT_per_isc_max  LowerLimit=ENG_CNT_per_isc_min
  Switch : Switch  Criteria=u2 > Threshold  Threshold=0.5
  per_isc_[%] : Outport
  wires:
  Switch/1 -> Saturation/1
  flag_idle_fb/1 -> Logical Operator1/1
  Gain/1 -> Switch/3
  Memory/1 -> Switch/1
  Saturation/1 -> per_isc_[%]/1, Memory/1
  del_omg_engine/1 -> Gain/1
  Logical Operator1/1 -> Switch/2

== system TRAMI_STEP_AT_vehicle_ver01_R2018b/Vehicle/ENG_CNT/Caliculate_Idle_Speed/Subsystem1 ==
  note: アイドル回転数時のFB
  omg_tgt_idle : Inport
  n_eng_rpm : Inport  Port=2
  per_throttle_base : Inport  Port=3
  flag_cutch_open : Inport  Port=4
  flag_IdleStop : Inport  Port=5
  Logical Operator : Logic  Operator=OR  AllPortsSameDT=off  OutDataTypeStr=boolean
  Logical Operator1 : Logic  Operator=NOT  AllPortsSameDT=off  OutDataTypeStr=boolean
  Logical Operator2 : Logic  Inputs=3  AllPortsSameDT=off  OutDataTypeStr=boolean
  Logical Operator4 : Logic  Operator=NOT  AllPortsSameDT=off  OutDataTypeStr=boolean
  Logical Operator5 : Logic  AllPortsSameDT=off  OutDataTypeStr=boolean
  Relational Operator : RelationalOperator  Operator=<  OutDataTypeStr=boolean  RndMeth=Nearest
  Relational Operator2 : RelationalOperator  Operator=>  OutDataTypeStr=boolean  RndMeth=Nearest
  per_throttle_isc_fb : Constant  Value=ENG_CNT_per_throttle_isc_fb
  flag_idle_fb : Outport
  wires:
  per_throttle_base/1 -> Relational Operator/1
  per_throttle_isc_fb/1 -> Relational Operator/2
  Relational Operator2/1 -> Logical Operator2/1
  Relational Operator/1 -> Logical Operator1/1, Logical Operator5/1
  Logical Operator1/1 -> Logical Operator2/2
  Logical Operator5/1 -> Logical Operator/2
  flag_cutch_open/1 -> Logical Operator2/3
  Logical Operator2/1 -> Logical Operator/1
  omg_tgt_idle/1 -> Relational Operator2/1
  n_eng_rpm/1 -> Relational Operator2/2
  flag_IdleStop/1 -> Logical Operator4/1
  Logical Operator4/1 -> Logical Operator5/2
  Logical Operator/1 -> flag_idle_fb/1

== system TRAMI_STEP_AT_vehicle_ver01_R2018b/Vehicle/ENG_PNT/Cal_FuelComsunption/Not_cal1 ==
  In1 : Inport
  Constant : Constant  Value=0
  Constant1 : Constant
  Switch : Switch  Criteria=u2 > Threshold  Threshold=0.5
  Out1 : Outport
  wires:
  Constant1/1 -> Switch/3
  Constant/1 -> Switch/1
  Switch/1 -> Out1/1
  In1/1 -> Switch/2

== system TRAMI_STEP_AT_vehicle_ver01_R2018b/Vehicle/ENG_PNT/Cal_FuelComsunption/Not_cal2 ==
  In1 : Inport
  Constant : Constant  Value=0
  Constant1 : Constant
  Switch : Switch  Criteria=u2 > Threshold  Threshold=0.5
  Out1 : Outport
  wires:
  In1/1 -> Switch/2
  Switch/1 -> Out1/1
  Constant/1 -> Switch/1
  Constant1/1 -> Switch/3

== system TRAMI_STEP_AT_vehicle_ver01_R2018b/Vehicle/ENG_PNT/Cal_trq_ENG_jiku/Not_cal ==
  In1 : Inport
  Constant : Constant  Value=0
  Constant1 : Constant
  Switch : Switch  Criteria=u2 > Threshold  Threshold=0.5
  Out1 : Outport
  wires:
  In1/1 -> Switch/2
  Switch/1 -> Out1/1
  Constant/1 -> Switch/1
  Constant1/1 -> Switch/3

== system TRAMI_STEP_AT_vehicle_ver01_R2018b/Vehicle/ENG_PNT/Cal_trq_ENG_jiku/Not_cal1 ==
  In1 : Inport
  Constant : Constant  Value=0
  Constant1 : Constant
  Switch : Switch  Criteria=u2 > Threshold  Threshold=0.5
  Out1 : Outport
  wires:
  Constant1/1 -> Switch/3
  Constant/1 -> Switch/1
  Switch/1 -> Out1/1
  In1/1 -> Switch/2

== system TRAMI_STEP_AT_vehicle_ver01_R2018b/Driver/Caliculate_Opeining_Accel/FF/Cal_M_ENG_jiku2/Subsystem ==
  In1 : Inport
  Constant1 : Constant  Value=0
  Switch : Switch  Criteria=u2 > Threshold  Threshold=0.1
  Out1 : Outport
  wires:
  Switch/1 -> Out1/1
  Constant1/1 -> Switch/3
  In1/1 -> Switch/2, Switch/1

== system TRAMI_STEP_AT_vehicle_ver01_R2018b/Vehicle/ALT_PNT/Subsystem/I_alt_cal/Cal_I_alt_P_control ==
  note: 目標電圧よりもオルタネータ電圧が低い場合電流をPI制御で出力
      | 高い場合は、電流を0とする
  V_delt_tgt : Inport
  Gain : Gain  Gain=ALT_PNT_Gain_Alt_v_del
  Transfer Fcn : TransferFcn  Denominator=[ALT_PNT_Tau_Alternator_V_tgt_s 1]
  I_alt_base : Outport
  wires:
  Gain/1 -> I_alt_base/1
  V_delt_tgt/1 -> Transfer Fcn/1
  Transfer Fcn/1 -> Gain/1

== system TRAMI_STEP_AT_vehicle_ver01_R2018b/Vehicle/ALT_PNT/Subsystem/I_alt_cal/Cal_I_alt_base ==
  note: 目標電圧よりもオルタネータ電圧が低い場合電流をPI制御で出力
      | 高い場合は、電流を0とする
  V_delt_tgt : Inport
  Constant : Constant  Value=0
  Gain : Gain  Gain=1/BT_PNT_Lo_R_lo_batt_ohm
  MinMax : MinMax  Function=max  Inputs=2
  Switch : Switch  Criteria=u2 > Threshold
  Transfer Fcn : TransferFcn  Denominator=[ALT_PNT_Tau_Alternator_V_tgt_s 1]
  I_alt_base : Outport
  wires:
  MinMax/1 -> I_alt_base/1
  Gain/1 -> Switch/1
  V_delt_tgt/1 -> Transfer Fcn/1
  Constant/1 -> MinMax/2, Switch/3
  Switch/1 -> MinMax/1
  Transfer Fcn/1 -> Switch/2, Gain/1
